simulink model "SimpleCardiovascularSystem_correctedv2"  (Simulink 6.6)
settings: Solver=ode45  StartTime=0.0  StopTime=10  RelTol=1e-3
libraries: simulink x1
settings Model: Creator=MXKana  LastModifiedBy=mxkana

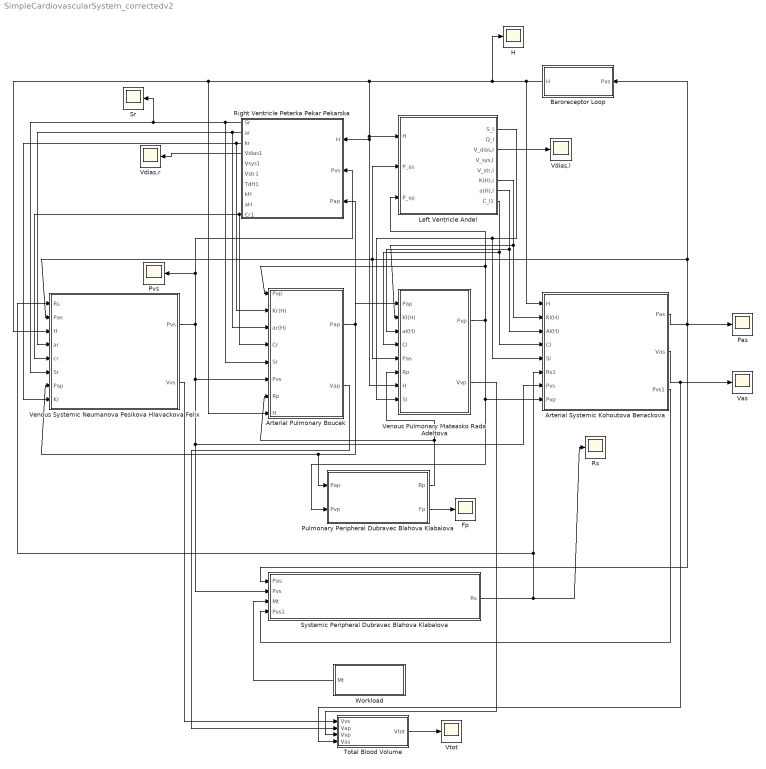
== system SimpleCardiovascularSystem_correctedv2 ==
  Arterial Pulmonary Boucek : Subsystem
  Arterial Systemic Kohoutova Benackova : Subsystem
  Baroreceptor Loop : Subsystem  Orientation=left
  Fp : Scope
      settings: YMin=1e+006  YMax=1e+007  SaveName=ScopeData5
  H : Scope
      settings: YMin=1e+006  YMax=1e+007  SaveName=ScopeData2
  Left Ventricle Andel : Subsystem
  Pas : Scope
      settings: YMin=-775  YMax=-475
  Pulmonary Peripheral Dubravec Blahova Klabalova : Subsystem
  Pvs : Scope
      settings: YMin=1e+006  YMax=1e+007  SaveName=ScopeData4
  Right Ventricle Peterka Pekar Pekarska : Subsystem  Orientation=left
  Rs : Scope
      settings: YMin=1e+006  YMax=1e+007  SaveName=ScopeData6
  Sr : Scope
      settings: YMin=1e+006  YMax=1e+007  SaveName=ScopeData7
  Systemic Peripheral Dubravec Blahova Klabalova : Subsystem
  Total Blood Volume : Subsystem
  Vas : Scope
  Vdias,l : Scope
      settings: YMin=1e+006  YMax=1e+007  SaveName=ScopeData9
  Vdias,r : Scope
      settings: YMin=1e+006  YMax=1e+007  SaveName=ScopeData8
  Venous Pulmonary Mateasko Rada Adeltova : Subsystem
  Venous Systemic Neumanova Pesikova Hlavackova Felix : Subsystem
  Vtot : Scope
      settings: YMin=1e+006  YMax=1e+007  SaveName=ScopeData3
  Workload : Subsystem  Orientation=left
  wires:
  Baroreceptor Loop/1(H) -> Arterial Systemic Kohoutova Benackova/1(H), Left Ventricle Andel/1(H), Venous Pulmonary Mateasko Rada Adeltova/7(H), Right Ventricle Peterka Pekar Pekarska/1(H), Venous Systemic Neumanova Pesikova Hlavackova Felix/3(H), Arterial Pulmonary Boucek/8(H), H/1
  Arterial Systemic Kohoutova Benackova/1(Pas) -> Baroreceptor Loop/1(Pas), Venous Pulmonary Mateasko Rada Adeltova/5(Pas), Venous Systemic Neumanova Pesikova Hlavackova Felix/2(Pas), Left Ventricle Andel/2(P_as), Systemic Peripheral Dubravec Blahova Klabalova/1(Pas), Pas/1
  Venous Systemic Neumanova Pesikova Hlavackova Felix/1(Pvs) -> Systemic Peripheral Dubravec Blahova Klabalova/2(Pvs), Arterial Systemic Kohoutova Benackova/7(Pvs), Arterial Pulmonary Boucek/6(Pvs), Right Ventricle Peterka Pekar Pekarska/2(Pvs), Pvs/1
  Arterial Pulmonary Boucek/1(Pap) -> Right Ventricle Peterka Pekar Pekarska/3(Pap), Pulmonary Peripheral Dubravec Blahova Klabalova/1(Pap), Venous Systemic Neumanova Pesikova Hlavackova Felix/7(Pap), Venous Pulmonary Mateasko Rada Adeltova/1(Pap)
  Venous Pulmonary Mateasko Rada Adeltova/1(Pvp) -> Arterial Systemic Kohoutova Benackova/8(Pvp), Pulmonary Peripheral Dubravec Blahova Klabalova/2(Pvp), Left Ventricle Andel/3(P_vp), Arterial Pulmonary Boucek/1(Pvp)
  Pulmonary Peripheral Dubravec Blahova Klabalova/1(Rp) -> Venous Pulmonary Mateasko Rada Adeltova/6(Rp), Arterial Pulmonary Boucek/7(Rp)
  Systemic Peripheral Dubravec Blahova Klabalova/1(Rs) -> Arterial Systemic Kohoutova Benackova/6(Rs1), Venous Systemic Neumanova Pesikova Hlavackova Felix/1(Rs), Rs/1
  Workload/1(Mt) -> Systemic Peripheral Dubravec Blahova Klabalova/3(Mt)
  Left Ventricle Andel/1(S_l) -> Venous Pulmonary Mateasko Rada Adeltova/8(Sl), Arterial Systemic Kohoutova Benackova/5(Sl)
  Left Ventricle Andel/6(K(H),l) -> Venous Pulmonary Mateasko Rada Adeltova/2(Kl(H)), Arterial Systemic Kohoutova Benackova/2(Kl(H))
  Left Ventricle Andel/7(a(H),l) -> Venous Pulmonary Mateasko Rada Adeltova/3(al(H)), Arterial Systemic Kohoutova Benackova/3(Al(H))
  Left Ventricle Andel/8(C_l1) -> Venous Pulmonary Mateasko Rada Adeltova/4(Cl), Arterial Systemic Kohoutova Benackova/4(Cl)
  Right Ventricle Peterka Pekar Pekarska/3(kr) -> Arterial Pulmonary Boucek/2(Kr(H)), Venous Systemic Neumanova Pesikova Hlavackova Felix/8(Kr)
  Right Ventricle Peterka Pekar Pekarska/2(ar) -> Arterial Pulmonary Boucek/3(ar(H)), Venous Systemic Neumanova Pesikova Hlavackova Felix/4(ar)
  Right Ventricle Peterka Pekar Pekarska/10(Cr1) -> Arterial Pulmonary Boucek/4(Cr), Venous Systemic Neumanova Pesikova Hlavackova Felix/5(cr)
  Right Ventricle Peterka Pekar Pekarska/1(Sr) -> Arterial Pulmonary Boucek/5(Sr), Venous Systemic Neumanova Pesikova Hlavackova Felix/6(Sr), Sr/1
  Venous Systemic Neumanova Pesikova Hlavackova Felix/2(Vvs) -> Total Blood Volume/1(Vvs)
  Arterial Pulmonary Boucek/2(Vap) -> Total Blood Volume/2(Vap)
  Venous Pulmonary Mateasko Rada Adeltova/2(Vvp) -> Total Blood Volume/3(Vvp)
  Arterial Systemic Kohoutova Benackova/2(Vas) -> Total Blood Volume/4(Vas), Vas/1
  Total Blood Volume/1(Vtot) -> Vtot/1
  Pulmonary Peripheral Dubravec Blahova Klabalova/2(Fp) -> Fp/1
  Right Ventricle Peterka Pekar Pekarska/4(Vdias1) -> Vdias,r/1
  Left Ventricle Andel/3(V_dias,l) -> Vdias,l/1
  Arterial Systemic Kohoutova Benackova/3(Pvs1) -> Systemic Peripheral Dubravec Blahova Klabalova/4(Pvs1)

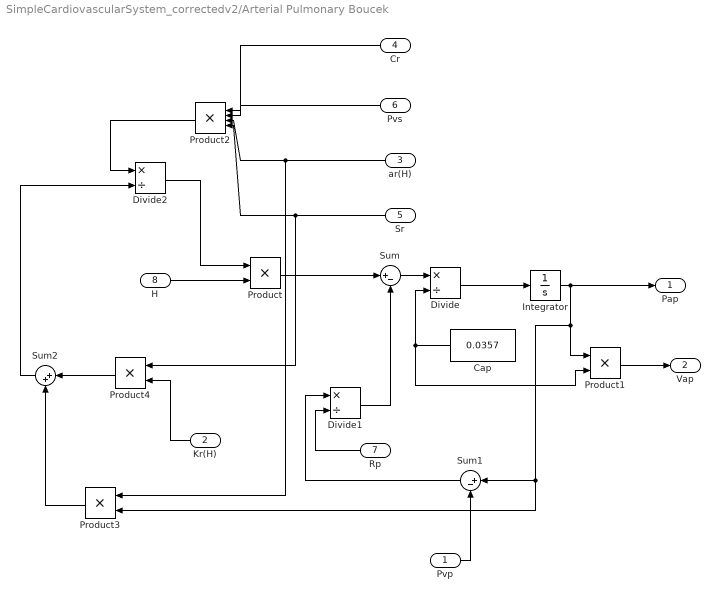
== system SimpleCardiovascularSystem_correctedv2/Arterial Pulmonary Boucek ==
  Pvp : Inport
  Kr(H) : Inport  Orientation=left  Port=2
  ar(H) : Inport  Orientation=left  Port=3
  Cr : Inport  Orientation=left  Port=4
  Sr : Inport  Orientation=left  Port=5
  Pvs : Inport  Orientation=left  Port=6
  Rp : Inport  Orientation=left  Port=7
  H : Inport  Port=8
  Cap : Constant  Orientation=left  Value=0.0357
  Divide : Product  Inputs=*/  OutScaling=2^-10
  Divide1 : Product  Inputs=*/  OutScaling=2^-10
  Divide2 : Product  Inputs=*/  OutScaling=2^-10
  Integrator : Integrator  InitialCondition=15
  Product : Product  RndMeth=Zero
  Product1 : Product  RndMeth=Zero
  Product2 : Product  Orientation=left  Inputs=4  RndMeth=Zero
  Product3 : Product  Orientation=left  RndMeth=Zero
  Product4 : Product  Orientation=left  RndMeth=Zero
  Sum : Sum  Inputs=|+-
  Sum1 : Sum  Orientation=left  Inputs=|+-
  Sum2 : Sum  Orientation=left  Inputs=|++
  Pap : Outport
  Vap : Outport  Port=2
  wires:
  Kr(H)/1 -> Product4/2
  Product3/1 -> Sum2/2
  Product4/1 -> Sum2/1
  Sum2/1 -> Divide2/2
  H/1 -> Product/2
  Divide2/1 -> Product/1
  Product2/1 -> Divide2/1
  Sr/1 -> Product4/1, Product2/4
  ar(H)/1 -> Product3/1, Product2/3
  Pvs/1 -> Product2/2
  Cr/1 -> Product2/1
  Product/1 -> Sum/1
  Divide1/1 -> Sum/2
  Rp/1 -> Divide1/2
  Sum1/1 -> Divide1/1
  Pvp/1 -> Sum1/2
  Product1/1 -> Vap/1
  Integrator/1 -> Pap/1, Product3/2, Sum1/1, Product1/1
  Divide/1 -> Integrator/1
  Cap/1 -> Product1/2, Divide/2
  Sum/1 -> Divide/1

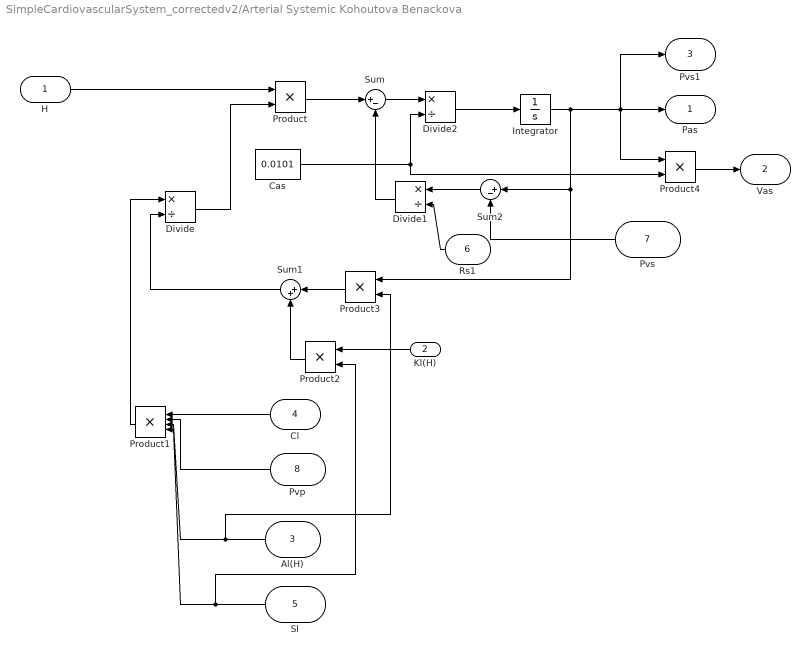
== system SimpleCardiovascularSystem_correctedv2/Arterial Systemic Kohoutova Benackova ==
  H : Inport
  Kl(H) : Inport  Orientation=left  Port=2
  Al(H) : Inport  Orientation=left  Port=3
  Cl : Inport  Orientation=left  Port=4
  Sl : Inport  Orientation=left  Port=5
  Rs1 : Inport  Orientation=left  Port=6
  Pvs : Inport  Orientation=left  Port=7
  Pvp : Inport  Orientation=left  Port=8
  Cas : Constant  Value=0.0101
  Divide : Product  Inputs=*/  OutScaling=2^-10
  Divide1 : Product  Orientation=left  Inputs=*/  OutScaling=2^-10
  Divide2 : Product  Inputs=*/  OutScaling=2^-10
  Integrator : Integrator  InitialCondition=105.5
  Product : Product  RndMeth=Zero
  Product1 : Product  Orientation=left  Inputs=4  RndMeth=Zero
  Product2 : Product  Orientation=left  RndMeth=Zero
  Product3 : Product  Orientation=left  RndMeth=Zero
  Product4 : Product  RndMeth=Zero
  Sum : Sum  Inputs=|+-
  Sum1 : Sum  Orientation=left  Inputs=|++
  Sum2 : Sum  Orientation=left  Inputs=|+-
  Pas : Outport
  Vas : Outport  Port=2
  Pvs1 : Outport  Port=3
  wires:
  Product4/1 -> Vas/1
  Cas/1 -> Product4/2, Divide2/2
  Sum/1 -> Divide2/1
  Divide2/1 -> Integrator/1
  Pvs/1 -> Sum2/2
  Integrator/1 -> Pas/1, Product4/1, Pvs1/1, Product3/1, Sum2/1
  Rs1/1 -> Divide1/2
  Sum2/1 -> Divide1/1
  Divide1/1 -> Sum/2
  Kl(H)/1 -> Product2/1
  Product2/1 -> Sum1/2
  Product3/1 -> Sum1/1
  Sl/1 -> Product2/2, Product1/4
  Al(H)/1 -> Product3/2, Product1/3
  Pvp/1 -> Product1/2
  Cl/1 -> Product1/1
  Sum1/1 -> Divide/2
  Product1/1 -> Divide/1
  Divide/1 -> Product/2
  Product/1 -> Sum/1
  H/1 -> Product/1

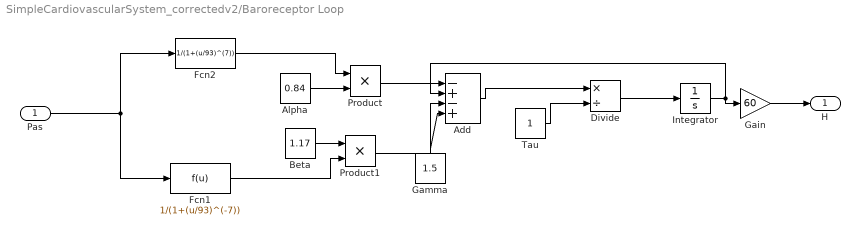
== system SimpleCardiovascularSystem_correctedv2/Baroreceptor Loop ==
  Pas : Inport
  Add : Sum  Inputs=-+-+  OutScaling=2^-10
  Alpha : Constant  Value=0.84
  Beta : Constant  Value=1.17
  Divide : Product  Inputs=*/  OutScaling=2^-10
  Fcn1 : Fcn  Expr=1/(1+(u/93)^(-7))
  Fcn2 : Fcn  Expr=1/(1+(u/93)^(7))
  Gain : Gain  Gain=60
  Gamma : Constant  Orientation=up  Value=1.5
  Integrator : Integrator  InitialCondition=0.2
  Product : Product  RndMeth=Zero
  Product1 : Product  RndMeth=Zero
  Tau : Constant
  H : Outport
  wires:
  Add/1 -> Divide/1
  Tau/1 -> Divide/2
  Divide/1 -> Integrator/1
  Integrator/1 -> Add/1, Gain/1
  Product/1 -> Add/2
  Product1/1 -> Add/3
  Beta/1 -> Product1/1
  Alpha/1 -> Product/2
  Gamma/1 -> Add/4
  Fcn1/1 -> Product1/2
  Fcn2/1 -> Product/1
  Pas/1 -> Fcn2/1, Fcn1/1
  Gain/1 -> H/1

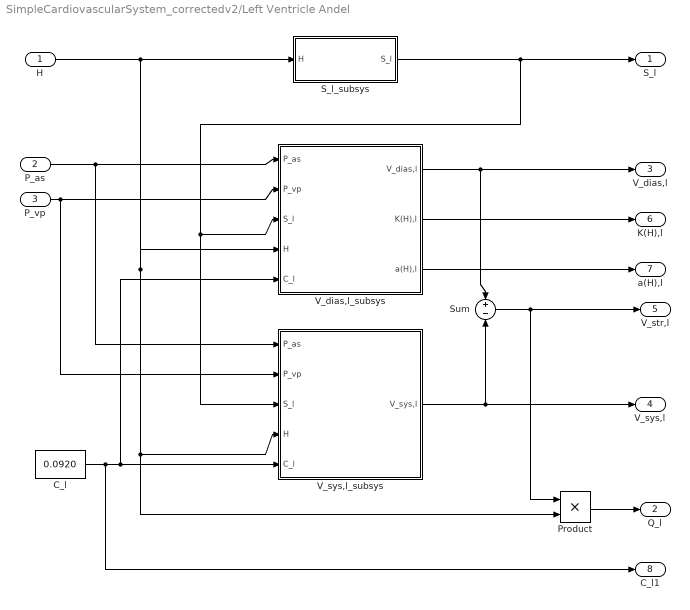
== system SimpleCardiovascularSystem_correctedv2/Left Ventricle Andel ==
  H : Inport
  P_as : Inport  Port=2
  P_vp : Inport  Port=3
  C_l : Constant  Value=0.0920
  Product : Product  RndMeth=Zero
  S_l_subsys : Subsystem
  Sum : Sum  Inputs=+-
  V_dias,l_subsys : Subsystem
  V_sys,l_subsys : Subsystem
  S_l : Outport
  Q_l : Outport  Port=2
  V_dias,l : Outport  Port=3
  V_sys,l : Outport  Port=4
  V_str,l : Outport  Port=5
  K(H),l : Outport  Port=6
  a(H),l : Outport  Port=7
  C_l1 : Outport  Port=8
  wires:
  Product/1 -> Q_l/1
  Sum/1 -> Product/1, V_str,l/1
  V_sys,l_subsys/1(V_sys,l) -> Sum/2, V_sys,l/1
  P_vp/1 -> V_sys,l_subsys/2(P_vp), V_dias,l_subsys/2(P_vp)
  P_as/1 -> V_sys,l_subsys/1(P_as), V_dias,l_subsys/1(P_as)
  V_dias,l_subsys/1(V_dias,l) -> Sum/1, V_dias,l/1
  S_l_subsys/1(S_l) -> V_sys,l_subsys/3(S_l), V_dias,l_subsys/3(S_l), S_l/1
  H/1 -> Product/2, V_sys,l_subsys/4(H), V_dias,l_subsys/4(H), S_l_subsys/1(H)
  C_l/1 -> V_sys,l_subsys/5(C_l), V_dias,l_subsys/5(C_l), C_l1/1
  V_dias,l_subsys/3(a(H),l) -> a(H),l/1
  V_dias,l_subsys/2(K(H),l) -> K(H),l/1

== system SimpleCardiovascularSystem_correctedv2/Pulmonary Peripheral Dubravec Blahova Klabalova ==
  Pap : Inport
  Pvp : Inport  Port=2
  Constant : Constant  Value=0.32
  Divide : Product  Inputs=*/  OutScaling=2^-10
  Subtract : Sum  Inputs=+-  OutScaling=2^-10
  Rp : Outport
  Fp : Outport  Port=2
  wires:
  Constant/1 -> Rp/1, Divide/2
  Pap/1 -> Subtract/1
  Pvp/1 -> Subtract/2
  Divide/1 -> Fp/1
  Subtract/1 -> Divide/1

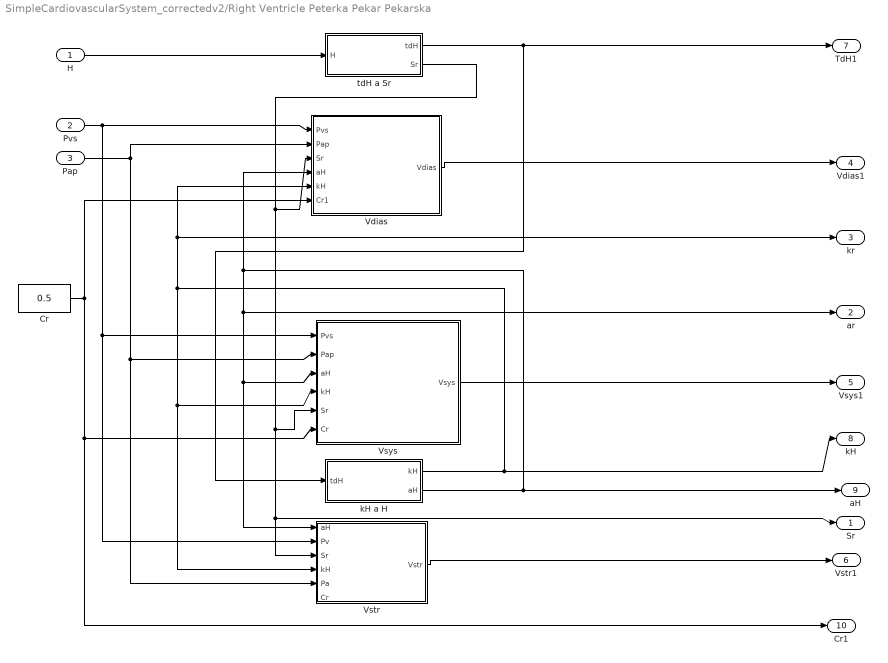
== system SimpleCardiovascularSystem_correctedv2/Right Ventricle Peterka Pekar Pekarska ==
  H : Inport
  Pvs : Inport  Port=2
  Pap : Inport  Port=3
  Cr : Constant  Value=0.5
  Vdias : Subsystem
  Vstr : Subsystem
  Vsys : Subsystem
  kH a H : Subsystem
  tdH a Sr : Subsystem
  Sr : Outport
  ar : Outport  Port=2
  kr : Outport  Port=3
  Vdias1 : Outport  Port=4
  Vsys1 : Outport  Port=5
  Vstr1 : Outport  Port=6
  TdH1 : Outport  Port=7
  kH : Outport  Port=8
  aH : Outport  Port=9
  Cr1 : Outport  Port=10
  wires:
  H/1 -> tdH a Sr/1(H)
  tdH a Sr/2(Sr) -> Vdias/3(Sr), Vstr/3(Sr), Sr/1, Vsys/5(Sr)
  tdH a Sr/1(tdH) -> kH a H/1(tdH), TdH1/1
  kH a H/2(aH) -> Vdias/4(aH), Vsys/3(aH), Vstr/1(aH), ar/1, aH/1
  kH a H/1(kH) -> Vsys/4(kH), Vstr/4(kH), Vdias/5(kH), kr/1, kH/1
  Vsys/1(Vsys) -> Vsys1/1
  Vstr/1(Vstr) -> Vstr1/1
  Pvs/1 -> Vdias/1(Pvs), Vsys/1(Pvs), Vstr/2(Pv)
  Pap/1 -> Vdias/2(Pap), Vsys/2(Pap), Vstr/5(Pa)
  Vdias/1(Vdias) -> Vdias1/1
  Cr/1 -> Vdias/6(Cr1), Vsys/6(Cr), Cr1/1

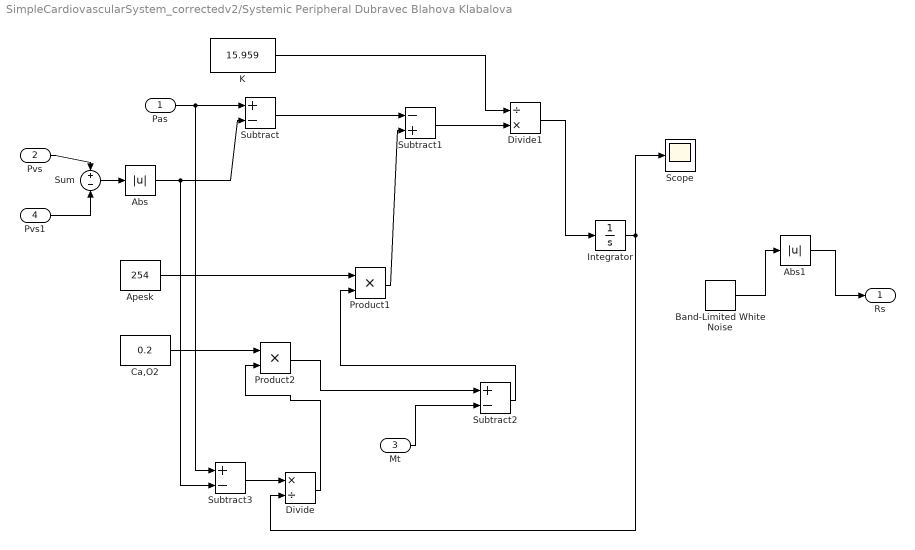
== system SimpleCardiovascularSystem_correctedv2/Systemic Peripheral Dubravec Blahova Klabalova ==
  Pas : Inport
      settings: BusObject=105.5
  Pvs : Inport  Port=2
      settings: BusObject=4
  Mt : Inport  Port=3
  Pvs1 : Inport  Port=4
  Abs : Abs
  Abs1 : Abs
  Apesk : Constant  Value=254
  Band-Limited White Noise : simulink/Sources/Band-Limited White Noise  SystemSampleTime=-1  Cov=[10]  Ts=0.1  seed=[23341]
  Ca,O2 : Constant  Value=0.2
  Divide : Product  Inputs=*/  OutScaling=2^-10
  Divide1 : Product  Inputs=/*  OutScaling=2^-10
  Integrator : Integrator  InitialCondition=9.5
  K : Constant  Value=15.959
  Product1 : Product  RndMeth=Zero
  Product2 : Product  RndMeth=Zero
  Scope : Scope
      settings: YMin=-1.75  YMax=1.75  SaveName=ScopeData10
  Subtract : Sum  Inputs=+-  OutScaling=2^-10
  Subtract1 : Sum  Inputs=-+  OutScaling=2^-10
  Subtract2 : Sum  Inputs=+-  OutScaling=2^-10
  Subtract3 : Sum  Inputs=+-  OutScaling=2^-10
  Sum : Sum  Inputs=+-
  Rs : Outport
  wires:
  Subtract3/1 -> Divide/1
  Divide/1 -> Product2/2
  Product2/1 -> Subtract2/1
  Ca,O2/1 -> Product2/1
  Integrator/1 -> Divide/2, Scope/1
  Divide1/1 -> Integrator/1
  Subtract1/1 -> Divide1/2
  Product1/1 -> Subtract1/2
  Subtract/1 -> Subtract1/1
  Subtract2/1 -> Product1/2
  Mt/1 -> Subtract2/2
  Apesk/1 -> Product1/1
  Pas/1 -> Subtract3/1, Subtract/1
  K/1 -> Divide1/1
  Pvs/1 -> Sum/1
  Pvs1/1 -> Sum/2
  Abs/1 -> Subtract/2, Subtract3/2
  Sum/1 -> Abs/1
  Band-Limited White Noise/1 -> Abs1/1
  Abs1/1 -> Rs/1

== system SimpleCardiovascularSystem_correctedv2/Total Blood Volume ==
  Vvs : Inport
  Vap : Inport  Port=2
  Vvp : Inport  Port=3
  Vas : Inport  Port=4
  Add : Sum  Inputs=++++  OutScaling=2^-10
  Vtot : Outport
  wires:
  Vvs/1 -> Add/1
  Vap/1 -> Add/2
  Vvp/1 -> Add/3
  Vas/1 -> Add/4
  Add/1 -> Vtot/1

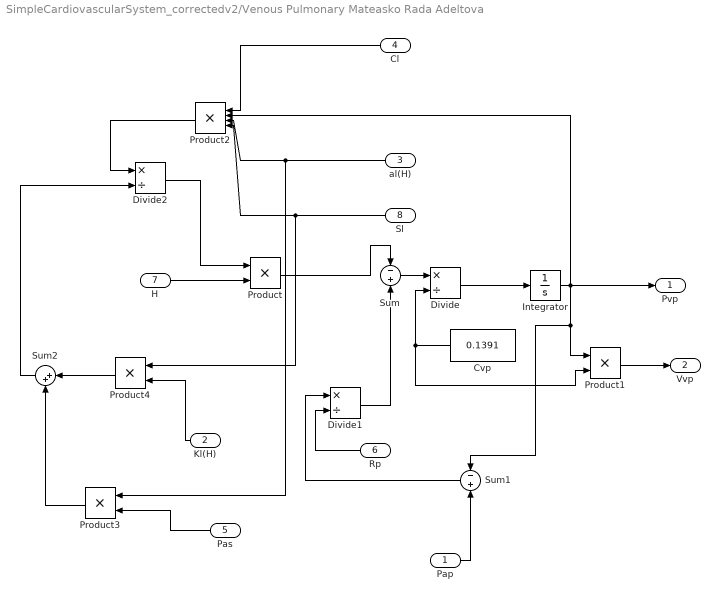
== system SimpleCardiovascularSystem_correctedv2/Venous Pulmonary Mateasko Rada Adeltova ==
  Pap : Inport
  Kl(H) : Inport  Orientation=left  Port=2
  al(H) : Inport  Orientation=left  Port=3
  Cl : Inport  Orientation=left  Port=4
  Pas : Inport  Orientation=left  Port=5
  Rp : Inport  Orientation=left  Port=6
  H : Inport  Port=7
  Sl : Inport  Orientation=left  Port=8
  Cvp : Constant  Orientation=left  Value=0.1391
  Divide : Product  Inputs=*/  OutScaling=2^-10
  Divide1 : Product  Inputs=*/  OutScaling=2^-10
  Divide2 : Product  Inputs=*/  OutScaling=2^-10
  Integrator : Integrator  InitialCondition=6
  Product : Product  RndMeth=Zero
  Product1 : Product  RndMeth=Zero
  Product2 : Product  Orientation=left  Inputs=4  RndMeth=Zero
  Product3 : Product  Orientation=left  RndMeth=Zero
  Product4 : Product  Orientation=left  RndMeth=Zero
  Sum : Sum  Inputs=-+
  Sum1 : Sum  Orientation=left  Inputs=-+
  Sum2 : Sum  Orientation=left  Inputs=|++
  Pvp : Outport
  Vvp : Outport  Port=2
  wires:
  Kl(H)/1 -> Product4/2
  Product3/1 -> Sum2/2
  Product4/1 -> Sum2/1
  Sum2/1 -> Divide2/2
  H/1 -> Product/2
  Divide2/1 -> Product/1
  Product2/1 -> Divide2/1
  Sl/1 -> Product4/1, Product2/4
  al(H)/1 -> Product3/1, Product2/3
  Cl/1 -> Product2/1
  Product/1 -> Sum/1
  Divide1/1 -> Sum/2
  Rp/1 -> Divide1/2
  Sum1/1 -> Divide1/1
  Pap/1 -> Sum1/2
  Product1/1 -> Vvp/1
  Integrator/1 -> Pvp/1, Product1/1, Sum1/1, Product2/2
  Divide/1 -> Integrator/1
  Cvp/1 -> Product1/2, Divide/2
  Sum/1 -> Divide/1
  Pas/1 -> Product3/2

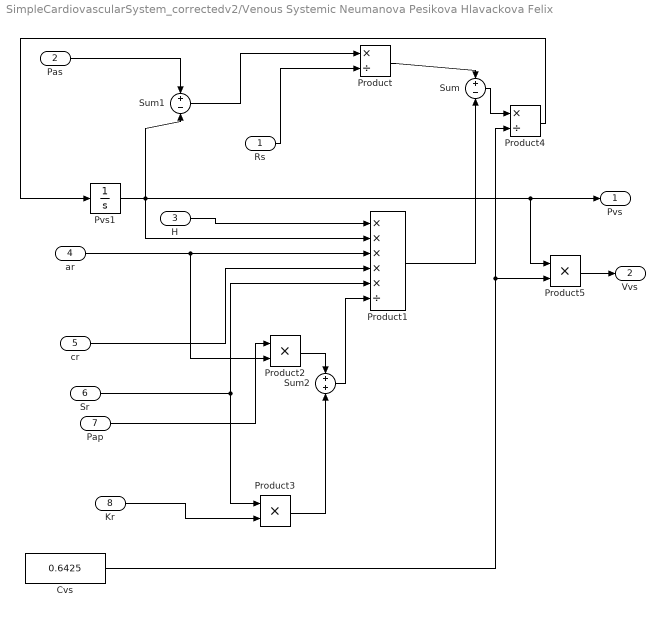
== system SimpleCardiovascularSystem_correctedv2/Venous Systemic Neumanova Pesikova Hlavackova Felix ==
  Rs : Inport
  Pas : Inport  Port=2
  H : Inport  Port=3
  ar : Inport  Port=4
  cr : Inport  Port=5
  Sr : Inport  Port=6
  Pap : Inport  Port=7
  Kr : Inport  Port=8
  Cvs : Constant  Value=0.6425
  Product : Product  Inputs=*/  RndMeth=Zero
  Product1 : Product  Inputs=*****/  RndMeth=Zero
  Product2 : Product  Inputs=**  RndMeth=Zero
  Product3 : Product  Inputs=**  RndMeth=Zero
  Product4 : Product  Inputs=*/  RndMeth=Zero
  Product5 : Product  Inputs=**  RndMeth=Zero
  Pvs1 : Integrator  InitialCondition=4
  Sum : Sum  Inputs=+-
  Sum1 : Sum  Inputs=+-
  Sum2 : Sum
  Pvs : Outport
  Vvs : Outport  Port=2
  wires:
  Product/1 -> Sum/1
  Rs/1 -> Product/2
  Pas/1 -> Sum1/1
  Sum1/1 -> Product/1
  Pvs1/1 -> Sum1/2, Product1/2, Pvs/1, Product5/1
  Product1/1 -> Sum/2
  H/1 -> Product1/1
  ar/1 -> Product1/3, Product2/2
  cr/1 -> Product1/4
  Sr/1 -> Product1/5, Product3/1
  Sum2/1 -> Product1/6
  Product2/1 -> Sum2/1
  Pap/1 -> Product2/1
  Product3/1 -> Sum2/2
  Kr/1 -> Product3/2
  Sum/1 -> Product4/1
  Cvs/1 -> Product4/2, Product5/2
  Product4/1 -> Pvs1/1
  Product5/1 -> Vvs/1

== system SimpleCardiovascularSystem_correctedv2/Workload ==
  Add : Sum  OutScaling=2^-10
  Mo : Constant  Value=0.35
  Product : Product  RndMeth=Zero
  Rau : Constant  Value=0.0011
  W : Constant  Value=75
  Mt : Outport
  wires:
  Rau/1 -> Product/1
  W/1 -> Product/2
  Product/1 -> Add/2
  Mo/1 -> Add/1
  Add/1 -> Mt/1

== system SimpleCardiovascularSystem_correctedv2/Left Ventricle Andel/S_l_subsys ==
  H : Inport
  Cr : Constant  Value=61
  S : Integrator  InitialCondition=61
  S' (t) : Integrator  InitialCondition=61
  Sum : Sum  Inputs=+--
  alfa_l : Gain  Orientation=left  Gain=31.592
  beta_l : Gain  Gain=25.065
  gama_l : Gain  Orientation=left  Gain=-1.332
  S_l : Outport
  wires:
  S/1 -> alfa_l/1
  H/1 -> beta_l/1
  alfa_l/1 -> Sum/2
  gama_l/1 -> Sum/3
  beta_l/1 -> Sum/1
  Sum/1 -> S' (t)/1
  S' (t)/1 -> gama_l/1, S/1
  Cr/1 -> S_l/1

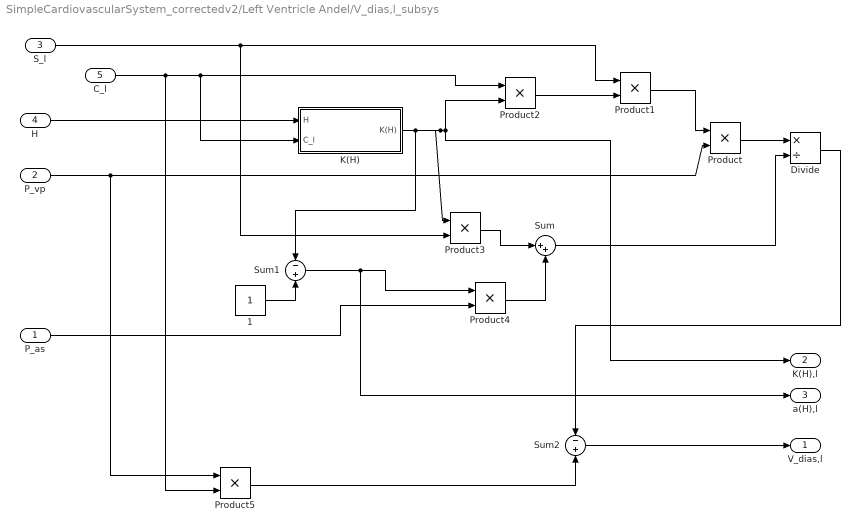
== system SimpleCardiovascularSystem_correctedv2/Left Ventricle Andel/V_dias,l_subsys ==
  P_as : Inport
  P_vp : Inport  Port=2
  S_l : Inport  Port=3
  H : Inport  Port=4
  C_l : Inport  Port=5
  1 : Constant
  Divide : Product  Inputs=*/  OutScaling=2^-10
  K(H) : Subsystem
  Product{,1..5} (6 alike) : Product  RndMeth=Zero
  Sum : Sum  Inputs=|++
  Sum1 : Sum  Inputs=-+
  Sum2 : Sum  Inputs=-+
  V_dias,l : Outport
  K(H),l : Outport  Port=2
  a(H),l : Outport  Port=3
  wires:
  P_as/1 -> Product4/2
  Sum1/1 -> Product4/1, a(H),l/1
  Sum2/1 -> V_dias,l/1
  Divide/1 -> Sum2/1
  Product5/1 -> Sum2/2
  H/1 -> K(H)/1(H)
  Sum/1 -> Divide/2
  1/1 -> Sum1/2
  Product4/1 -> Sum/2
  Product3/1 -> Sum/1
  K(H)/1(K(H)) -> Sum1/1, Product3/1, Product2/2, K(H),l/1
  Product/1 -> Divide/1
  Product2/1 -> Product1/2
  C_l/1 -> K(H)/2(C_l), Product2/1, Product5/2
  Product1/1 -> Product/1
  S_l/1 -> Product3/2, Product1/1
  P_vp/1 -> Product5/1, Product/2

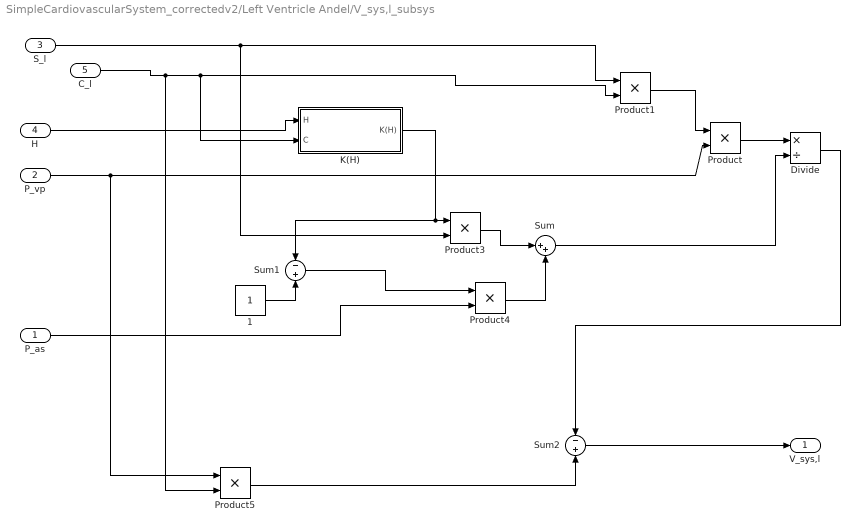
== system SimpleCardiovascularSystem_correctedv2/Left Ventricle Andel/V_sys,l_subsys ==
  P_as : Inport
  P_vp : Inport  Port=2
  S_l : Inport  Port=3
  H : Inport  Port=4
  C_l : Inport  Port=5
  1 : Constant
  Divide : Product  Inputs=*/  OutScaling=2^-10
  K(H) : Subsystem
  Product{,1,3..5} (5 alike) : Product  RndMeth=Zero
  Sum : Sum  Inputs=|++
  Sum1 : Sum  Inputs=-+
  Sum2 : Sum  Inputs=-+
  V_sys,l : Outport
  wires:
  K(H)/1(K(H)) -> Sum1/1, Product3/1
  P_as/1 -> Product4/2
  Sum1/1 -> Product4/1
  Sum2/1 -> V_sys,l/1
  Divide/1 -> Sum2/1
  Product5/1 -> Sum2/2
  H/1 -> K(H)/1(H)
  Sum/1 -> Divide/2
  1/1 -> Sum1/2
  Product4/1 -> Sum/2
  Product3/1 -> Sum/1
  Product/1 -> Divide/1
  C_l/1 -> Product1/2, K(H)/2(C), Product5/2
  Product1/1 -> Product/1
  S_l/1 -> Product3/2, Product1/1
  P_vp/1 -> Product5/1, Product/2

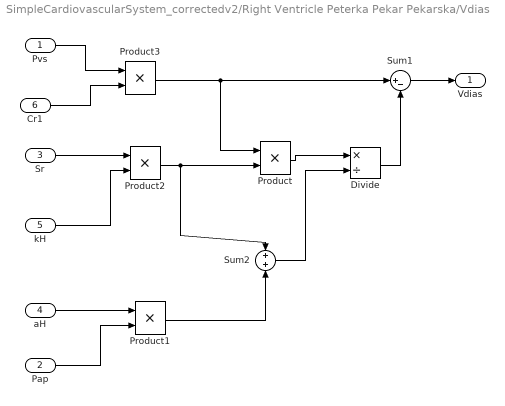
== system SimpleCardiovascularSystem_correctedv2/Right Ventricle Peterka Pekar Pekarska/Vdias ==
  Pvs : Inport
  Pap : Inport  Port=2
  Sr : Inport  Port=3
  aH : Inport  Port=4
  kH : Inport  Port=5
  Cr1 : Inport  Port=6
  Divide : Product  Inputs=*/  OutScaling=2^-10
  Product{,1..3} (4 alike) : Product  RndMeth=Zero
  Sum1 : Sum  Inputs=|+-
  Sum2 : Sum
  Vdias : Outport
  wires:
  Pvs/1 -> Product3/1
  Product3/1 -> Sum1/1, Product/1
  Sum1/1 -> Vdias/1
  Divide/1 -> Sum1/2
  Product/1 -> Divide/1
  aH/1 -> Product1/1
  Pap/1 -> Product1/2
  Sr/1 -> Product2/1
  kH/1 -> Product2/2
  Product2/1 -> Product/2, Sum2/1
  Product1/1 -> Sum2/2
  Sum2/1 -> Divide/2
  Cr1/1 -> Product3/2

== system SimpleCardiovascularSystem_correctedv2/Right Ventricle Peterka Pekar Pekarska/Vstr ==
  aH : Inport
  Pv : Inport  Port=2
  Sr : Inport  Port=3
  kH : Inport  Port=4
  Pa : Inport  Port=5
  Cr : Inport  Port=6
  Divide : Product  Inputs=*/  OutScaling=2^-10
  Product : Product  Inputs=3  RndMeth=Zero
  Product1 : Product  RndMeth=Zero
  Product2 : Product  RndMeth=Zero
  Product3 : Product  RndMeth=Zero
  Sum : Sum  Inputs=|++
  Vstr : Outport
  wires:
  aH/1 -> Product1/1, Product3/1
  Pv/1 -> Product/2
  Sr/1 -> Product/3, Product2/1
  Pa/1 -> Product1/2
  kH/1 -> Product2/2
  Product1/1 -> Sum/1
  Product2/1 -> Sum/2
  Product/1 -> Divide/1
  Sum/1 -> Divide/2
  Divide/1 -> Vstr/1
  Cr/1 -> Product3/2
  Product3/1 -> Product/1

== system SimpleCardiovascularSystem_correctedv2/Right Ventricle Peterka Pekar Pekarska/Vsys ==
  Pvs : Inport
  Pap : Inport  Port=2
  aH : Inport  Port=3
  kH : Inport  Port=4
  Sr : Inport  Port=5
  Cr : Inport  Port=6
  Divide1 : Product  Inputs=*/  OutScaling=2^-10
  Product{,1..3} (4 alike) : Product  RndMeth=Zero
  Sum3 : Sum  Inputs=|+-
  Sum4 : Sum
  Vsys : Outport
  wires:
  Pvs/1 -> Product2/1
  Product2/1 -> Sum3/1, Product3/1
  Sum3/1 -> Vsys/1
  Divide1/1 -> Sum3/2
  Product3/1 -> Divide1/1
  aH/1 -> Product/1
  Pap/1 -> Product/2
  Sr/1 -> Product1/1, Product3/2
  Product/1 -> Sum4/2
  Sum4/1 -> Divide1/2
  Product1/1 -> Sum4/1
  kH/1 -> Product1/2
  Cr/1 -> Product2/2

== system SimpleCardiovascularSystem_correctedv2/Right Ventricle Peterka Pekar Pekarska/kH a H ==
  tdH : Inport
  Constant : Constant
  Constant1 : Constant
  Divide : Product  Inputs=*/  OutScaling=2^-10
  Math Function : Math  SaturateOnIntegerOverflow=on
  Product : Product  RndMeth=Zero
  Rp : Constant  Value=0.32
  Sum : Sum  Inputs=|-+
  c : Gain  Gain=-1
  kH : Outport
  aH : Outport  Port=2
  wires:
  Math Function/1 -> kH/1, Sum/1
  Product/1 -> Math Function/1
  Rp/1 -> c/1
  c/1 -> Divide/2
  Constant/1 -> Divide/1
  Divide/1 -> Product/1
  tdH/1 -> Product/2
  Constant1/1 -> Sum/2
  Sum/1 -> aH/1

== system SimpleCardiovascularSystem_correctedv2/Right Ventricle Peterka Pekar Pekarska/tdH a Sr ==
  H : Inport
  Alfa r : Gain  Orientation=left  Gain=28.342
  Beta r : Gain  Gain=1.416
  Cr : Constant  Value=4
  Fcn : Fcn  Expr=(1/(u^0.5))*(1/(u^0.5)-0.0516)
  Gamma r : Gain  Orientation=left  Gain=-2.045
  Integrator : Integrator  InitialCondition=4
  Integrator1 : Integrator  InitialCondition=4
  Sum : Sum  Inputs=|+--
  tdH : Outport
  Sr : Outport  Port=2
  wires:
  Integrator1/1 -> Integrator/1, Gamma r/1  "dS/dt"
  Gamma r/1 -> Sum/3
  H/1 -> Beta r/1, Fcn/1
  Sum/1 -> Integrator1/1  "ddS/dt"
  Beta r/1 -> Sum/1
  Fcn/1 -> tdH/1
  Integrator/1 -> Alfa r/1  "S"
  Alfa r/1 -> Sum/2
  Cr/1 -> Sr/1

== system SimpleCardiovascularSystem_correctedv2/Left Ventricle Andel/V_dias,l_subsys/K(H) ==
  H : Inport
  C_l : Inport  Port=2
  1 : Constant
  Divide : Product  Inputs=*/  OutScaling=2^-10
  Fcn : Fcn  Expr=exp(-u)
  Product : Product  RndMeth=Zero
  Product1 : Product  RndMeth=Zero
  R : Constant  Value=0.32
  t_d(H) : Subsystem
  K(H) : Outport
  wires:
  Fcn/1 -> K(H)/1
  Product1/1 -> Fcn/1
  t_d(H)/1(t_d(H)) -> Product1/1
  Divide/1 -> Product1/2
  1/1 -> Divide/1
  Product/1 -> Divide/2
  R/1 -> Product/2
  C_l/1 -> Product/1
  H/1 -> t_d(H)/1(H)

== system SimpleCardiovascularSystem_correctedv2/Left Ventricle Andel/V_sys,l_subsys/K(H) ==
  H : Inport
  C : Inport  Port=2
  1 : Constant
  Divide : Product  Inputs=*/  OutScaling=2^-10
  Fcn : Fcn  Expr=exp(-u)
  Product : Product  RndMeth=Zero
  Product1 : Product  RndMeth=Zero
  R : Constant  Value=0.32
  t_d(H) : Subsystem
  K(H) : Outport
  wires:
  Fcn/1 -> K(H)/1
  Product1/1 -> Fcn/1
  t_d(H)/1(t_d(H)) -> Product1/1
  Divide/1 -> Product1/2
  1/1 -> Divide/1
  Product/1 -> Divide/2
  R/1 -> Product/2
  C/1 -> Product/1
  H/1 -> t_d(H)/1(H)

== system SimpleCardiovascularSystem_correctedv2/Left Ventricle Andel/V_dias,l_subsys/K(H)/t_d(H) ==
  H : Inport
  1 : Constant
  Divide : Product  Inputs=*/  OutScaling=2^-10
  Fcn : Fcn  Expr=u^(1/2)
  Product : Product  RndMeth=Zero
  Sum : Sum  Inputs=+-
  k : Constant  Value=0.0516
  t_d(H) : Outport
  wires:
  k/1 -> Sum/2
  Sum/1 -> Product/2
  Product/1 -> t_d(H)/1
  Divide/1 -> Sum/1, Product/1
  1/1 -> Divide/1
  Fcn/1 -> Divide/2
  H/1 -> Fcn/1

== system SimpleCardiovascularSystem_correctedv2/Left Ventricle Andel/V_sys,l_subsys/K(H)/t_d(H) ==
  H : Inport
  1 : Constant
  Divide : Product  Inputs=*/  OutScaling=2^-10
  Fcn : Fcn  Expr=u^(1/2)
  Product : Product  RndMeth=Zero
  Sum : Sum  Inputs=+-
  k : Constant  Value=0.0516
  t_d(H) : Outport
  wires:
  Sum/1 -> Product/2
  k/1 -> Sum/2
  Product/1 -> t_d(H)/1
  Divide/1 -> Sum/1, Product/1
  1/1 -> Divide/1
  Fcn/1 -> Divide/2
  H/1 -> Fcn/1
